simulink model "NCS_MPC_QoS_tele"  (Simulink 7.1)
settings: Solver=ode45  StartTime=0.0  StopTime=duration_time  RelTol=1e-3
undefined symbols (not defined in the file or in its folder): Af, Bf, Cf, De, Df, fH, kD_slave, KDh_force, KDh_pos, Ke, kI_slave, KIh_force, KIh_pos, kP_slave, KPh_force, KPh_pos, Me, ssAmh, ssAs, ssBmh, ssBs, ssCmh, ssCs, ssDmh, ssDs, Ts, xE
libraries: simulink x3
settings Model: Creator=riccardo  LastModifiedBy=riccardo

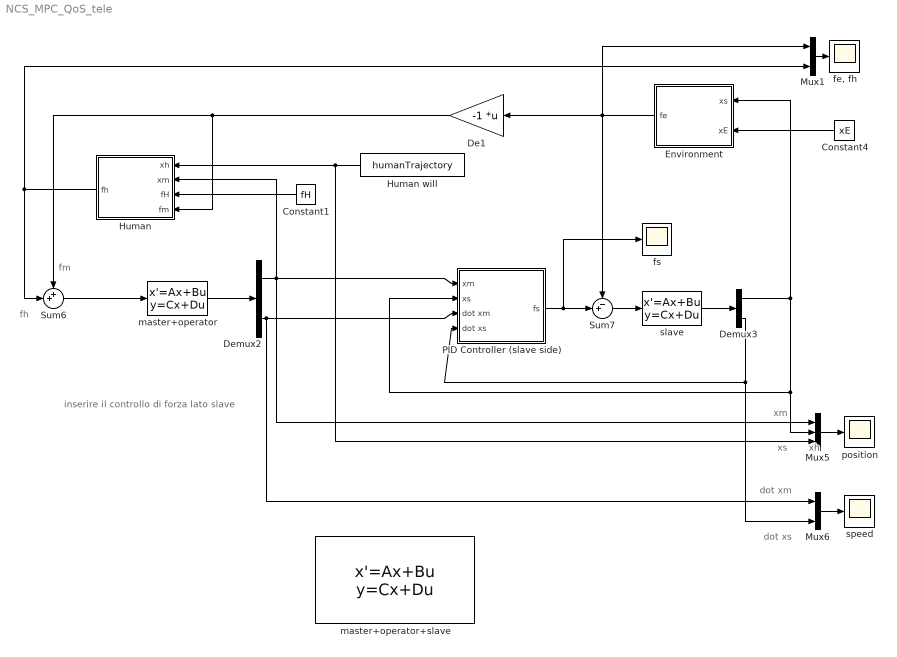
== system NCS_MPC_QoS_tele ==
  note: xm
  note: xs
  note: dot xm
  note: dot xs
  note: fm
  note: fh
  note: xh
  note: inserire il controllo
      | di forza lato slave
  Constant1 : Constant  Orientation=left  Value=fH  OutDataType=sfix(16)  OutScaling=2^0
  Constant4 : Constant  Orientation=left  Value=xE  OutDataType=sfix(16)  OutScaling=2^0
  De1 : Gain  Orientation=left  Gain=-1  Multiplication=Matrix(K*u)  ParameterDataType=sfix(16)  ParameterScaling=2^0  OutDataType=sfix(16)  OutScaling=2^0
  Demux2 : Demux  Outputs=2
  Demux3 : Demux  Outputs=2
  Environment : Subsystem  Orientation=left
  Human : Subsystem  Orientation=left
  Human will : FromWorkspace  Orientation=left  VariableName=humanTrajectory  SampleTime=0
  Mux1 : Mux  Inputs=2
  Mux5 : Mux  Inputs=3
  Mux6 : Mux  Inputs=2
  PID Controller (slave side) : Subsystem
  Sum6 : Sum  Inputs=++|  OutDataType=sfix(16)  OutScaling=2^0
  Sum7 : Sum  Inputs=-+|  OutDataType=sfix(16)  OutScaling=2^0
  "fe, fh" : Scope
      settings: YMin=-1  YMax=1  SaveName=ScopeData2
  fs : Scope
      settings: YMin=-1  YMax=1
  master+operator : StateSpace  A=ssAmh  B=ssBmh  C=ssCmh  D=ssDmh
  master+operator+slave : StateSpace  A=Af  B=Bf  C=Cf  D=Df
  position : Scope
      settings: SaveName=ScopeData3
  slave : StateSpace  A=ssAs  B=ssBs  C=ssCs  D=ssDs
  speed : Scope
      settings: YMin=-0.25  YMax=0.3  SaveName=ScopeData4
  wires:
  Environment/1(fe) -> Sum7/1, Mux1/1, De1/1
  Human/1(fh) -> Sum6/2, Mux1/2
  Sum6/1 -> master+operator/1
  master+operator/1 -> Demux2/1
  Demux2/1 -> Mux5/1, PID Controller (slave side)/1(xm), Human/2(xm)
  Demux2/2 -> Mux6/1, PID Controller (slave side)/3(dot xm)
  Sum7/1 -> slave/1
  PID Controller (slave side)/1(fs) -> Sum7/2, fs/1
  slave/1 -> Demux3/1
  Demux3/2 -> Mux6/2, PID Controller (slave side)/4(dot xs)
  Demux3/1 -> Mux5/2, PID Controller (slave side)/2(xs), Environment/1(xs)
  Mux5/1 -> position/1
  Mux6/1 -> speed/1
  Constant4/1 -> Environment/2(xE)
  Constant1/1 -> Human/3(fH)
  Human will/1 -> Human/1(xh), Mux5/3
  Mux1/1 -> "fe, fh"/1
  De1/1 -> Human/4(fm), Sum6/1

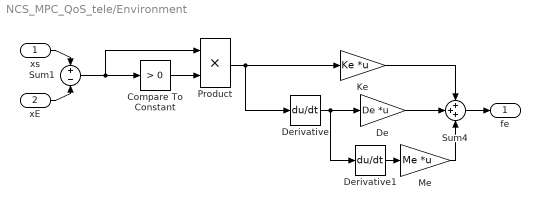
== system NCS_MPC_QoS_tele/Environment ==
  xs : Inport
  xE : Inport  Port=2
  Compare To Constant : simulink/Logic and Bit Operations/Compare To Constant  SystemSampleTime=-1  relop=>  const=0  LogicOutDataTypeMode=uint8  ZeroCross=off
  De : Gain  Gain=De  Multiplication=Matrix(K*u)  ParameterDataType=sfix(16)  ParameterScaling=2^0  OutDataType=sfix(16)  OutScaling=2^0
  Derivative : Derivative
  Derivative1 : Derivative
  Ke : Gain  Gain=Ke  Multiplication=Matrix(K*u)  ParameterDataType=sfix(16)  ParameterScaling=2^0  OutDataType=sfix(16)  OutScaling=2^0
  Me : Gain  Gain=Me  Multiplication=Matrix(K*u)  ParameterDataType=sfix(16)  ParameterScaling=2^0  OutDataType=sfix(16)  OutScaling=2^0
  Product : Product  OutDataType=sfix(16)  OutScaling=2^0  RndMeth=Zero
  Sum1 : Sum  Inputs=+|-  OutDataType=sfix(16)  OutScaling=2^0
  Sum4 : Sum  Inputs=+++  OutDataType=sfix(16)  OutScaling=2^0
  fe : Outport
  wires:
  Compare To Constant/1 -> Product/2
  Sum1/1 -> Compare To Constant/1, Product/1
  Product/1 -> Ke/1, Derivative/1
  Derivative/1 -> De/1, Derivative1/1
  Derivative1/1 -> Me/1
  Ke/1 -> Sum4/1
  De/1 -> Sum4/2
  Me/1 -> Sum4/3
  xs/1 -> Sum1/1
  xE/1 -> Sum1/2
  Sum4/1 -> fe/1

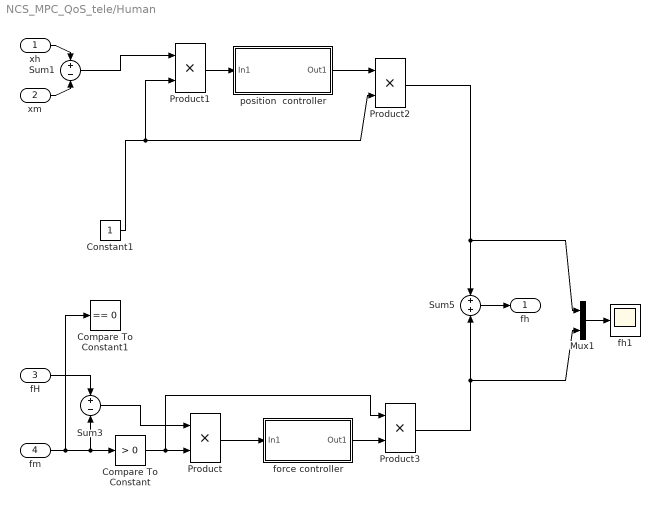
== system NCS_MPC_QoS_tele/Human ==
  xh : Inport
  xm : Inport  Port=2
  fH : Inport  Port=3
  fm : Inport  Port=4
  Compare To Constant : simulink/Logic and Bit Operations/Compare To Constant  SystemSampleTime=-1  relop=>  const=0  LogicOutDataTypeMode=uint8  ZeroCross=off
  Compare To Constant1 : simulink/Logic and Bit Operations/Compare To Constant  SystemSampleTime=-1  relop===  const=0  LogicOutDataTypeMode=uint8  ZeroCross=off
  Constant1 : Constant  OutDataType=sfix(16)  OutScaling=2^0
  Mux1 : Mux  Inputs=2
  Product{,1..3} (4 alike) : Product  OutDataType=sfix(16)  OutScaling=2^0  RndMeth=Zero
  Sum1 : Sum  Inputs=+|-  OutDataType=sfix(16)  OutScaling=2^0
  Sum3 : Sum  Inputs=+|-  OutDataType=sfix(16)  OutScaling=2^0
  Sum5 : Sum  Inputs=+|+  OutDataType=sfix(16)  OutScaling=2^0
  fh1 : Scope
      settings: YMin=-1  YMax=1
  force controller : Subsystem
  position  controller : Subsystem
  fh : Outport
  wires:
  xh/1 -> Sum1/1
  xm/1 -> Sum1/2
  fm/1 -> Sum3/2, Compare To Constant/1, Compare To Constant1/1
  fH/1 -> Sum3/1
  Compare To Constant/1 -> Product/2, Product3/1
  Sum3/1 -> Product/1
  Constant1/1 -> Product1/2, Product2/2
  Sum1/1 -> Product1/1
  Product1/1 -> position  controller/1(In1)
  Product/1 -> force controller/1(In1)
  position  controller/1(Out1) -> Product2/1
  force controller/1(Out1) -> Product3/2
  Product3/1 -> Mux1/2, Sum5/2
  Product2/1 -> Sum5/1, Mux1/1
  Sum5/1 -> fh/1
  Mux1/1 -> fh1/1

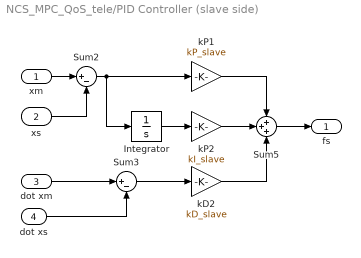
== system NCS_MPC_QoS_tele/PID Controller (slave side) ==
  xm : Inport
  xs : Inport  Port=2
  dot xm : Inport  Port=3
  dot xs : Inport  Port=4
  Integrator : Integrator
  Sum2 : Sum  Inputs=|+-  OutDataType=sfix(16)  OutScaling=2^0
  Sum3 : Sum  Inputs=|+-  OutDataType=sfix(16)  OutScaling=2^0
  Sum5 : Sum  Inputs=+++  OutDataType=sfix(16)  OutScaling=2^0
  kD2 : Gain  Gain=kD_slave  ParameterDataType=sfix(16)  ParameterScaling=2^0  OutDataType=sfix(16)  OutScaling=2^0  SampleTime=Ts
  kP1 : Gain  Gain=kP_slave  ParameterDataType=sfix(16)  ParameterScaling=2^0  OutDataType=sfix(16)  OutScaling=2^0  SampleTime=Ts
  kP2 : Gain  Gain=kI_slave  ParameterDataType=sfix(16)  ParameterScaling=2^0  OutDataType=sfix(16)  OutScaling=2^0  SampleTime=Ts
  fs : Outport
  wires:
  Sum2/1 -> kP1/1, Integrator/1
  Sum3/1 -> kD2/1
  kP1/1 -> Sum5/1
  xm/1 -> Sum2/1
  xs/1 -> Sum2/2
  dot xm/1 -> Sum3/1
  dot xs/1 -> Sum3/2
  Sum5/1 -> fs/1
  kD2/1 -> Sum5/3
  kP2/1 -> Sum5/2
  Integrator/1 -> kP2/1

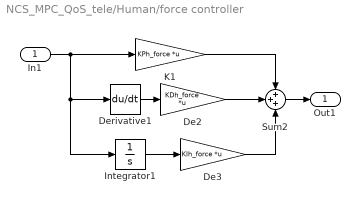
== system NCS_MPC_QoS_tele/Human/force controller ==
  In1 : Inport
  De2 : Gain  Gain=KDh_force  Multiplication=Matrix(K*u)  ParameterDataType=sfix(16)  ParameterScaling=2^0  OutDataType=sfix(16)  OutScaling=2^0
  De3 : Gain  Gain=KIh_force  Multiplication=Matrix(K*u)  ParameterDataType=sfix(16)  ParameterScaling=2^0  OutDataType=sfix(16)  OutScaling=2^0
  Derivative1 : Derivative
  Integrator1 : Integrator
  K1 : Gain  Gain=KPh_force  Multiplication=Matrix(K*u)  ParameterDataType=sfix(16)  ParameterScaling=2^0  OutDataType=sfix(16)  OutScaling=2^0
  Sum2 : Sum  Inputs=+++  OutDataType=sfix(16)  OutScaling=2^0
  Out1 : Outport
  wires:
  In1/1 -> Integrator1/1, Derivative1/1, K1/1
  Derivative1/1 -> De2/1
  K1/1 -> Sum2/1
  De2/1 -> Sum2/2
  De3/1 -> Sum2/3
  Integrator1/1 -> De3/1
  Sum2/1 -> Out1/1

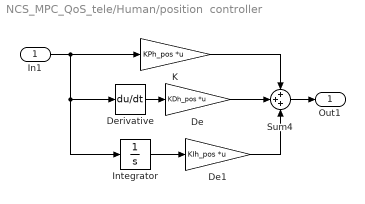
== system NCS_MPC_QoS_tele/Human/position  controller ==
  In1 : Inport
  De : Gain  Gain=KDh_pos  Multiplication=Matrix(K*u)  ParameterDataType=sfix(16)  ParameterScaling=2^0  OutDataType=sfix(16)  OutScaling=2^0
  De1 : Gain  Gain=KIh_pos  Multiplication=Matrix(K*u)  ParameterDataType=sfix(16)  ParameterScaling=2^0  OutDataType=sfix(16)  OutScaling=2^0
  Derivative : Derivative
  Integrator : Integrator
  K : Gain  Gain=KPh_pos  Multiplication=Matrix(K*u)  ParameterDataType=sfix(16)  ParameterScaling=2^0  OutDataType=sfix(16)  OutScaling=2^0
  Sum4 : Sum  Inputs=+++  OutDataType=sfix(16)  OutScaling=2^0
  Out1 : Outport
  wires:
  In1/1 -> Integrator/1, Derivative/1, K/1
  Derivative/1 -> De/1
  K/1 -> Sum4/1
  De/1 -> Sum4/2
  De1/1 -> Sum4/3
  Integrator/1 -> De1/1
  Sum4/1 -> Out1/1
